simulink model "Equ7_2_1"  (Simulink 8.9)
settings: Solver=ode45  StartTime=0.0  StopTime=20.0  RelTol=1e-3  EnableMultiTasking=on
settings Model: SuppressorTable=22 serialization::archive 11 0 6 0 0 0 0 0  Creator=Anita Enmark  LastModifiedBy=pechorin
settings OptimizationCC: ExpressionDepthLimit=2147483647  InitFltsAndDblsToZero=on
settings DebuggingCC: SaveWithParameterizedLinksMsg=none  SignalResolutionControl=TryResolveAllWithWarning  SolverPrmCheckMsg=warning
settings GRTTargetCC: TargetFcnLib=ansi_tfl_tmw.mat

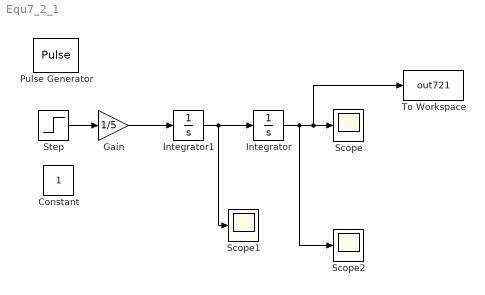
== system Equ7_2_1 ==
  Constant : Constant
  Gain : Gain  Gain=1/5
  Integrator : Integrator
  Integrator1 : Integrator
  Pulse Generator : DiscretePulseGenerator  PulseType=Time based  PulseWidth=50
  Scope : Scope
  Scope1 : Scope
  Scope2 : Scope
  Step : Step  SampleTime=0
  To Workspace : ToWorkspace  VariableName=out721  SaveFormat=Timeseries  SampleTime=-1
  wires:
  Integrator1/1 -> Scope1/1, Integrator/1
  Integrator/1 -> Scope2/1, Scope/1, To Workspace/1
  Step/1 -> Gain/1
  Gain/1 -> Integrator1/1
